simulink model "S_RS_B_Custom_Model"  (R2024b)
settings: Solver=ode23t  StartTime=0.0  StopTime=6*3600  MaxStep=0.03  RelTol=1e-6
model workspace (MAT data in the model file):
  C048A = [-4.646 -4.60016161616 -4.553 -4.506 -4.459 -4.41180808081 -4.36496969697 -4.31813131313 -4.27129292929 -4.22445454545 -4.17761616162 -4.13077777778 ... (100 elements, 100x1)]
  C25C = [-4.6365 -4.58998989899 -4.54347979798 -4.49604545455 -4.44945959596 -4.40294949495 -4.35593939394 -4.30893939394 -4.26241919192 -4.21540909091 -4.16848484848 -4.12155555556 ... (100 elements, 100x1)]
  C40C = [-4.693 -4.64635858586 -4.59905555556 -4.55133333333 -4.50411111111 -4.45679292929 -4.40916666667 -4.36194444444 -4.31472222222 -4.26727272727 -4.21977777778 -4.17244444444 ... (100 elements, 100x1)]
  C48A = [-4.565 -4.51971717172 -4.47343434343 -4.42715151515 -4.38086868687 -4.335 -4.289 -4.243 -4.19673737374 -4.15045454545 -4.10417171717 -4.058 ... (100 elements, 100x1)]
  C55C = [-4.736 -4.68873737374 -4.64097474747 -4.59321212121 -4.54544444444 -4.49718686869 -4.44942424242 -4.40166161616 -4.3538989899 -4.30613636364 -4.25837373737 -4.21061111111 ... (100 elements, 100x1)]
  C72A = [-4.552 -4.50695959596 -4.46091919192 -4.41487878788 -4.36983838384 -4.3237979798 -4.27775757576 -4.23171717172 -4.18567676768 -4.13963636364 -4.0935959596 -4.04755555556 ... (100 elements, 100x1)]
  C96A = [-4.554 -4.5084040404 -4.4625 -4.4165 -4.3705 -4.32467676768 -4.27863636364 -4.23257575758 -4.18651515152 -4.14045454545 -4.09439393939 -4.04838888889 ... (100 elements, 100x1)]
  I048A = [-0.48 -0.48 -0.48 -0.48 -0.48 -0.48 -0.48 -0.48 -0.48 -0.48 -0.48 -0.48 ... (100 elements, 100x1)]
  I48A = [-4.792 -4.792 -4.792 -4.792 -4.792 -4.792 -4.792 -4.792 -4.792 -4.792 -4.792 -4.792 ... (100 elements, 100x1)]
  I72A = [-7.19 -7.191 -7.191 -7.191 -7.191 -7.191 -7.191 -7.191 -7.191 -7.191 -7.191 -7.191 ... (100 elements, 100x1)]
  I96A = [-9.591 -9.591 -9.591 -9.591 -9.591 -9.591 -9.591 -9.591 -9.591 -9.591 -9.591 -9.591 ... (100 elements, 100x1)]
  Param : Simulink.Parameter (value not decoded)
  RT048 = [0 0 0 0 0 0 0 0 0 0 0 0 ... (100 elements, 100x1)]
  RT048A = [0 0 0 0 0 0 0 0 0 0 0 0 ... (100 elements, 100x1)]
  RT48A = [0 0.0119433061837 0.0174343602975 0.0201725097385 0.0218841166254 0.022368931384 0.0223984418475 0.0231362034367 0.0227462437396 0.0224237365306 0.0230708588388 0.0242533852717 ... (100 elements, 100x1)]
  RT72A = [0 0.0122979200993 0.0175935407475 0.020202020202 0.0216937838965 0.0225267555263 0.0230549129172 0.0237221330254 0.0239187873731 0.0241969128077 0.0252237294373 0.0266691388928 ... (100 elements, 100x1)]
  RT96A = [0 0.0106302309931 0.015521179894 0.0181246307302 0.0198249832282 0.0208391916243 0.0215479790081 0.0224110566619 0.0227069990911 0.0230234784504 0.0239687038248 0.0253072903996 ... (100 elements, 100x1)]
  SOC01C = [0 0.00986620401171 0.0200172191132 0.0301334481274 0.0402496771416 0.0504072146345 0.0604886575614 0.0705701004883 0.0806515434152 0.0907329863421 0.100814429269 0.110895872196 ... (100 elements, 100x1)]
  SOC15C = [0 0.00989464060642 0.0200089648684 0.0301232891303 0.0400179297367 0.0501322539987 0.0602465782606 0.0703609025226 0.0804752267845 0.0905895510465 0.100703875308 0.11081819957 ... (100 elements, 100x1)]
  SOC1C = [0 0.00991956807948 0.0200581942093 0.0301968203392 0.0403354464691 0.0503833515882 0.0604600219058 0.0705366922234 0.0806708929381 0.090809519068 0.100948145198 0.111062431544 ... (100 elements, 100x1)]
  SOC25C = [0 0.0100312953758 0.0200625907517 0.0302932266698 0.0403408614344 0.0503721568102 0.0605112921515 0.0706482489077 0.0806817228687 0.0908208582101 0.100941475578 0.111063182238 ... (100 elements, 100x1)]
  SOC2C = [0 0.0100122880097 0.020092226614 0.030193236715 0.040294246816 0.050356441002 0.0604663233122 0.0705806417269 0.0806949601416 0.0908092785563 0.100923596971 0.111025716098 ... (100 elements, 100x1)]
  SOC40C = [0 0.00993850716842 0.0200179937022 0.03018680304 0.04024907072 0.0503317857888 0.0604801477378 0.0705424154178 0.0806046830978 0.090715378804 0.100835760116 0.110921703719 ... (100 elements, 100x1)]
  SOC55C = [0 0.00997943966694 0.0200644536582 0.0301494676495 0.040235548048 0.0504250699563 0.0605100839476 0.0705950979388 0.0806801119301 0.0907651259214 0.100850139913 0.110935153904 ... (100 elements, 100x1)]
  T25C = [297.946805556 297.946193603 297.929952862 297.907583333 297.879161616 297.864882155 297.845863636 297.84875 297.844378788 297.852901515 297.87439899 297.893138889 ... (100 elements, 100x1)]
  T40C = [312.783611111 312.799016835 312.779327441 312.709037879 312.764760943 312.775969697 312.760472222 312.812088384 312.770179293 312.777401515 312.764757576 312.816768519 ... (100 elements, 100x1)]
  T55C = [327.602916667 327.628770202 327.629694444 327.60230303 327.617340909 327.627280303 327.630606061 327.639113636 327.603484848 327.641583333 327.626977273 327.647388889 ... (100 elements, 100x1)]
  V048A = [2.5 2.68851515152 2.80367676768 2.88551515152 2.951 3.00419191919 3.05003030303 3.09186868687 3.124 3.153 3.18438383838 3.21722222222 ... (100 elements, 100x1)]
  V25C = [2.4995 2.68887878788 2.80454040404 2.88553030303 2.95054040404 3.00379292929 3.04906060606 3.09057070707 3.13208080808 3.17309090909 3.21251515152 3.24794444444 ... (100 elements, 100x1)]
  V40C = [2.499 2.68894444444 2.80844444444 2.89090909091 2.95538888889 3.00911111111 3.05384848485 3.09348989899 3.13214646465 3.17127272727 3.21022222222 3.24738888889 ... (100 elements, 100x1)]
  V48A = [2.5 2.63128282828 2.72013131313 2.78884848485 2.84613131313 2.897 2.9426969697 2.981 3.015 3.04554545455 3.07382828283 3.101 ... (100 elements, 100x1)]
  V55C = [2.499 2.68891414141 2.80855050505 2.89028787879 2.95405050505 3.00636868687 3.05007575758 3.08772222222 3.12348989899 3.1595 3.19588888889 3.2315 ... (100 elements, 100x1)]
  V72A = [2.5 2.60008080808 2.67716161616 2.74024242424 2.795 2.8422020202 2.88424242424 2.92128282828 2.952 2.979 3.003 3.02544444444 ... (100 elements, 100x1)]
  V96A = [2.5 2.58656060606 2.65481313131 2.71168181818 2.76085858586 2.80432323232 2.84336363636 2.87692424242 2.90621717172 2.93218181818 2.9545 2.9745 ... (100 elements, 100x1)]
  t_CHG_25C = [18010 17847.8787879 17665.7575758 17483.6363636 17301.5151515 17119.3939394 16952.2727273 16770.1515152 16588.030303 16420.9090909 16238.7878788 16056.6666667 ... (100 elements, 100x1)]
  t_CHG_40C = [14605 14477.2727273 14329.5454545 14181.8181818 14049.0909091 13901.3636364 13768.6363636 13620.9090909 13473.1818182 13325.4545455 13177.7272727 13030 ... (100 elements, 100x1)]
  t_CHG_55C = [17190 17046.0606061 16872.1212121 16719.5454545 16554.2424242 16380.3030303 16206.3636364 16032.4242424 15858.4848485 15684.5454545 15510.6060606 15336.6666667 ... (100 elements, 100x1)]
libraries: BatteryEstimators x1
(part 2 of 2)

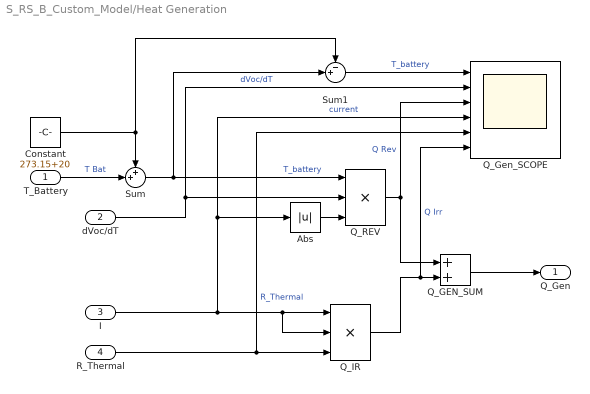
== system S_RS_B_Custom_Model/Heat Generation ==
  T_Battery : Inport
  dVoc/dT : Inport  Port=2
  I : Inport  Port=3
  R_Thermal : Inport  Port=4
  Abs : Abs  SaturateOnIntegerOverflow=off
  Constant : Constant  Value=273.15+20
  Q_GEN_SUM : Sum
  Q_Gen_SCOPE : Scope  NumInputPorts=6
  Q_IR : Product  Inputs=3
  Q_REV : Product  Inputs=3
  Sum : Sum  Inputs=++|
  Sum1 : Sum  Inputs=-+|
  Q_Gen : Outport
  wires:
  Q_REV/1 -> Q_GEN_SUM/1, Q_Gen_SCOPE/3  "Q Rev"
  I/1 -> Q_IR/2, Q_IR/1, Abs/1, Q_Gen_SCOPE/4  "current"
  R_Thermal/1 -> Q_IR/3, Q_Gen_SCOPE/5  "R_Thermal"
  Q_IR/1 -> Q_Gen_SCOPE/6, Q_GEN_SUM/2  "Q Irr"
  dVoc/dT/1 -> Q_REV/2, Q_Gen_SCOPE/2  "dVoc/dT"
  Q_GEN_SUM/1 -> Q_Gen/1
  Abs/1 -> Q_REV/3
  T_Battery/1 -> Sum/2  "T Bat"
  Constant/1 -> Sum1/1, Sum/1
  Sum/1 -> Sum1/2, Q_REV/1  "T_battery"
  Sum1/1 -> Q_Gen_SCOPE/1  "T_battery"

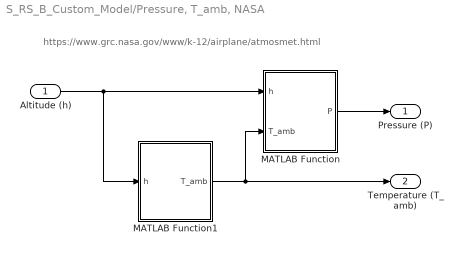
== system S_RS_B_Custom_Model/Pressure, T_amb, NASA ==
  note: https://www.grc.nasa.gov/www/k-12/airplane/atmosmet.html
  Altitude (h) : Inport
  MATLAB Function : MATLAB Function  TreatAsAtomicUnit=on
  MATLAB Function1 : MATLAB Function  TreatAsAtomicUnit=on
  Pressure (P) : Outport
  Temperature (T_amb) : Outport  Port=2
  wires:
  MATLAB Function1/1(T_amb) -> MATLAB Function/2(T_amb), Temperature (T_amb)/1
  MATLAB Function/1(P) -> Pressure (P)/1
  Altitude (h)/1 -> MATLAB Function/1(h), MATLAB Function1/1(h)

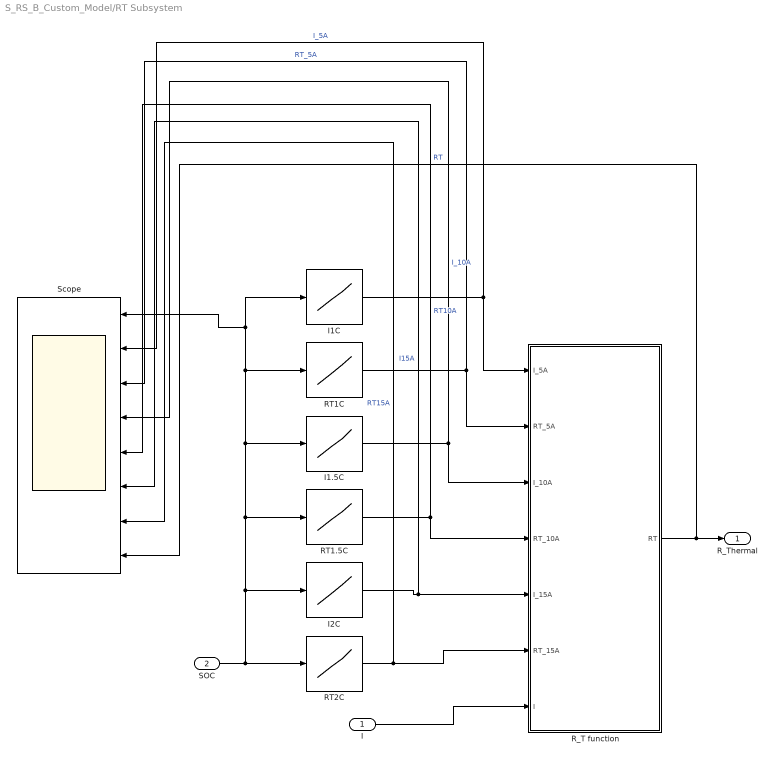
== system S_RS_B_Custom_Model/RT Subsystem ==
  I : Inport
  SOC : Inport  Port=2
  I1.5C : Lookup_n-D  NumberOfTableDimensions=1  BreakpointsForDimension1=SOC15C  Table=I72A  InternalRulePriority=Speed  RndMeth=Simplest
  I1C : Lookup_n-D  NumberOfTableDimensions=1  BreakpointsForDimension1=SOC1C  Table=I48A  InternalRulePriority=Speed  RndMeth=Simplest
  I2C : Lookup_n-D  NumberOfTableDimensions=1  BreakpointsForDimension1=SOC2C  Table=I96A  InternalRulePriority=Speed  RndMeth=Simplest
  RT1.5C : Lookup_n-D  NumberOfTableDimensions=1  BreakpointsForDimension1=SOC15C  Table=RT72A  InternalRulePriority=Speed  RndMeth=Simplest
  RT1C : Lookup_n-D  NumberOfTableDimensions=1  BreakpointsForDimension1=SOC1C  Table=RT48A  InternalRulePriority=Speed  RndMeth=Simplest
  RT2C : Lookup_n-D  NumberOfTableDimensions=1  BreakpointsForDimension1=SOC2C  Table=RT96A  InternalRulePriority=Speed  RndMeth=Simplest
  R_T function : MATLAB Function  TreatAsAtomicUnit=on
  Scope : Scope  NumInputPorts=8
  R_Thermal : Outport
  wires:
  R_T function/1(RT) -> Scope/8, R_Thermal/1  "RT"
  I/1 -> R_T function/7(I)
  SOC/1 -> RT1C/1, I1C/1, Scope/1, I1.5C/1, RT1.5C/1, I2C/1, RT2C/1
  I1C/1 -> R_T function/1(I_5A), Scope/2  "I_5A"
  RT1C/1 -> R_T function/2(RT_5A), Scope/3  "RT_5A"
  I1.5C/1 -> R_T function/3(I_10A), Scope/4  "I_10A"
  RT1.5C/1 -> R_T function/4(RT_10A), Scope/5  "RT10A"
  I2C/1 -> Scope/6, R_T function/5(I_15A)  "I15A"
  RT2C/1 -> Scope/7, R_T function/6(RT_15A)  "RT15A"

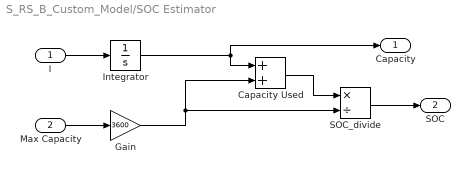
== system S_RS_B_Custom_Model/SOC Estimator ==
  I : Inport
  Max Capacity : Inport  Port=2
  Capacity Used : Sum
  Gain : Gain  Gain=3600
  Integrator : Integrator
  SOC_divide : Product  Inputs=*/
  Capacity : Outport
  SOC : Outport  Port=2
  wires:
  Capacity Used/1 -> SOC_divide/1
  SOC_divide/1 -> SOC/1
  I/1 -> Integrator/1
  Max Capacity/1 -> Gain/1
  Gain/1 -> SOC_divide/2, Capacity Used/2
  Integrator/1 -> Capacity Used/1, Capacity/1

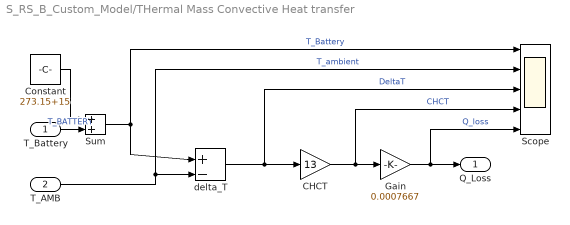
== system S_RS_B_Custom_Model/THermal Mass Convective Heat transfer ==
  T_Battery : Inport
  T_AMB : Inport  Port=2
  CHCT : Gain  Gain=13
  Constant : Constant  Value=273.15+15
  Gain : Gain  Gain=0.0007667
  Scope : Scope  NumInputPorts=5
  Sum : Sum  Inputs=+|+
  delta_T : Sum  Inputs=+|-
  Q_Loss : Outport
  wires:
  T_AMB/1 -> Scope/2, delta_T/2  "T_ambient"
  delta_T/1 -> Scope/3, CHCT/1  "DeltaT"
  CHCT/1 -> Scope/4, Gain/1  "CHCT"
  Gain/1 -> Scope/5, Q_Loss/1  "Q_loss"
  T_Battery/1 -> Sum/2  "T_BATTERY"
  Sum/1 -> delta_T/1, Scope/1  "T_Battery"
  Constant/1 -> Sum/1

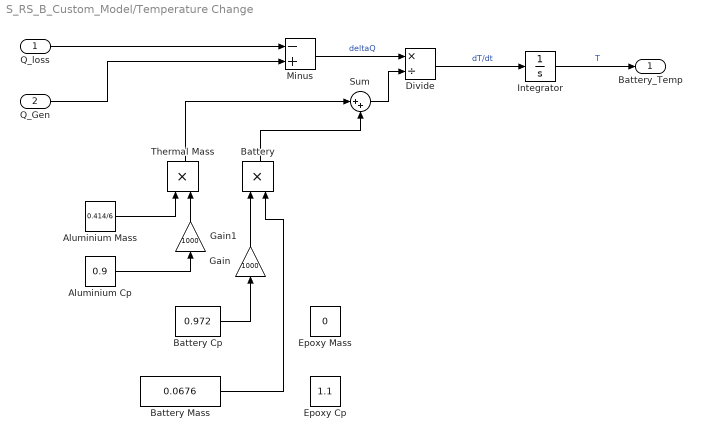
== system S_RS_B_Custom_Model/Temperature Change ==
  Q_loss : Inport
  Q_Gen : Inport  Port=2
  Aluminium Cp : Constant  Value=0.9  VectorParams1D=off
  Aluminium Mass : Constant  Value=0.414/6  VectorParams1D=off
  Battery : Product  OutDataTypeStr=double
  Battery Cp : Constant  Value=0.972  VectorParams1D=off
  Battery Mass : Constant  Value=0.0676  VectorParams1D=off
  Divide : Product  Inputs=*/
  Epoxy Cp : Constant  Value=1.1  VectorParams1D=off
  Epoxy Mass : Constant  Value=0  VectorParams1D=off
  Gain : Gain  Gain=1000
  Gain1 : Gain  Gain=1000
  Integrator : Integrator
  Minus : Sum  Inputs=-+
  Sum : Sum  Inputs=|++
  Thermal Mass : Product  OutDataTypeStr=double
  Battery_Temp : Outport
  wires:
  Integrator/1 -> Battery_Temp/1  "T"
  Battery/1 -> Sum/2
  Divide/1 -> Integrator/1  "dT/dt"
  Minus/1 -> Divide/1  "deltaQ"
  Sum/1 -> Divide/2
  Battery Cp/1 -> Gain/1
  Aluminium Cp/1 -> Gain1/1
  Aluminium Mass/1 -> Thermal Mass/1
  Q_loss/1 -> Minus/1
  Q_Gen/1 -> Minus/2
  Battery Mass/1 -> Battery/2
  Gain/1 -> Battery/1
  Thermal Mass/1 -> Sum/1
  Gain1/1 -> Thermal Mass/2

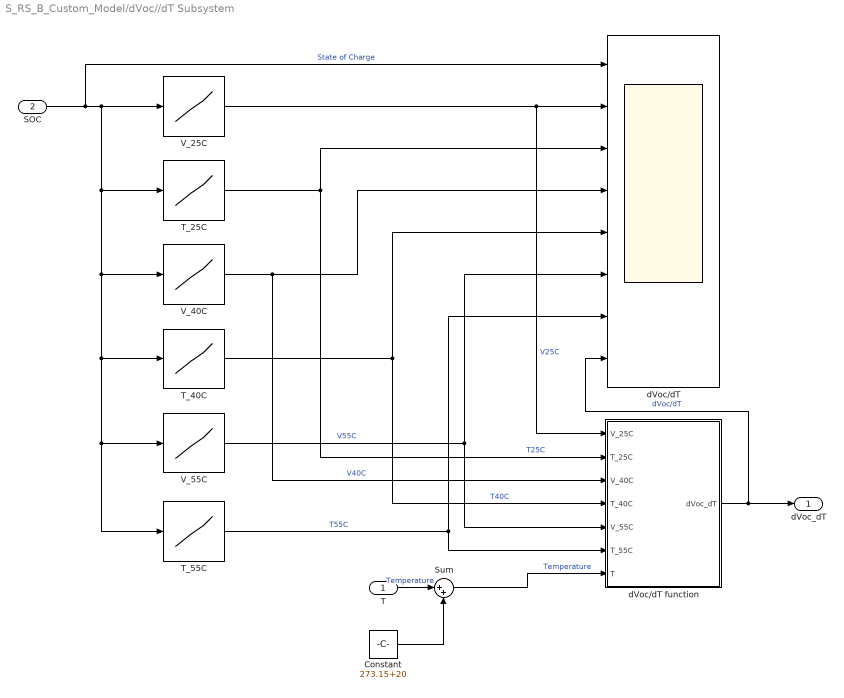
== system S_RS_B_Custom_Model/dVoc//dT Subsystem ==
  T : Inport
  SOC : Inport  Port=2
  Constant : Constant  Value=273.15+20
  Sum : Sum  Inputs=|++
  T_25C : Lookup_n-D  NumberOfTableDimensions=1  BreakpointsForDimension1=SOC25C  Table=T25C  InternalRulePriority=Speed  RndMeth=Simplest  SupportTunableSize=on
  T_40C : Lookup_n-D  NumberOfTableDimensions=1  BreakpointsForDimension1=SOC40C  Table=T40C  InternalRulePriority=Speed  RndMeth=Simplest  SupportTunableSize=on
  T_55C : Lookup_n-D  NumberOfTableDimensions=1  BreakpointsForDimension1=SOC55C  Table=T55C  InternalRulePriority=Speed  RndMeth=Simplest  SupportTunableSize=on
  V_25C : Lookup_n-D  NumberOfTableDimensions=1  BreakpointsForDimension1=SOC25C  Table=V25C  InternalRulePriority=Speed  RndMeth=Simplest  SupportTunableSize=on
  V_40C : Lookup_n-D  NumberOfTableDimensions=1  BreakpointsForDimension1=SOC40C  Table=V40C  InternalRulePriority=Speed  RndMeth=Simplest  SupportTunableSize=on
  V_55C : Lookup_n-D  NumberOfTableDimensions=1  BreakpointsForDimension1=SOC55C  Table=V55C  InternalRulePriority=Speed  RndMeth=Simplest  SupportTunableSize=on
  dVoc/dT : Scope  NumInputPorts=8
  dVoc/dT function : MATLAB Function  TreatAsAtomicUnit=on
  dVoc_dT : Outport
  wires:
  Sum/1 -> dVoc/dT function/7(T)  "Temperature"
  dVoc/dT function/1(dVoc_dT) -> dVoc/dT/8, dVoc_dT/1  "dVoc/dT"
  V_25C/1 -> dVoc/dT function/1(V_25C), dVoc/dT/2  "V25C"
  T_25C/1 -> dVoc/dT function/2(T_25C), dVoc/dT/3  "T25C"
  V_40C/1 -> dVoc/dT function/3(V_40C), dVoc/dT/4  "V40C"
  T_40C/1 -> dVoc/dT function/4(T_40C), dVoc/dT/5  "T40C"
  V_55C/1 -> dVoc/dT function/5(V_55C), dVoc/dT/6  "V55C"
  T_55C/1 -> dVoc/dT/7, dVoc/dT function/6(T_55C)  "T55C"
  SOC/1 -> dVoc/dT/1, T_55C/1, V_55C/1, T_40C/1, V_40C/1, T_25C/1, V_25C/1  "State of Charge"
  T/1 -> Sum/1  "Temperature"
  Constant/1 -> Sum/2

== matlab function S_RS_B_Custom_Model/RT Subsystem/R_T function ==
  data: I_5A input; RT_5A input; I_10A input; RT output; RT_10A input; I_15A input; RT_15A input; I input
function RT = fcn(I_5A,RT_5A, I_10A,RT_10A, I_15A,RT_15A, I)
    
    %Current Index
    a= I_5A;
    b= I_10A;
    c= I_15A;

    %Lagrange polynomial 
  
    Rt_1C = RT_5A .* (I-b) .* (I-c)  ./ ((a-b) .* (a-c) ); 
    Rt_2C = RT_10A .* (I-a) .* (I-c) ./ ((b-a) .* (b-c) );
    Rt_3C = RT_15A .* (I-a) .* (I-b) ./ ((c-a) .* (c-b) );

    RT = Rt_1C + Rt_2C + Rt_3C; 

end

== matlab function S_RS_B_Custom_Model/dVoc//dT Subsystem/dVoc//dT function ==
  data: V_25C input; T_25C input; V_40C input; T_40C input; V_55C input; T_55C input; T input; dVoc_dT output
function dVoc_dT = fcn(V_25C,T_25C, V_40C,T_40C, V_55C,T_55C,  T)

    dVoc_25C = V_25C .* (2*T - T_40C - T_55C) / ( (T_25C - T_40C ) * (T_25C - T_55C) ); 
    dVoc_40C = V_40C .* (2*T - T_25C - T_55C) / ( (T_40C - T_25C ) * (T_40C - T_55C ) ); 
    dVoc_55C = V_55C .* (2*T - T_25C - T_40C) / ( (T_55C - T_25C ) * (T_55C - T_40C ) );

    %Output
    dVoc_dT = double(dVoc_25C + dVoc_40C + dVoc_55C); 
    
end

== matlab function S_RS_B_Custom_Model/Cell Voltage/V function ==
  data: I_0_5A input; V_0_5A input; I_5A input; V_5A input; I_10A input; V output; V_10A input; I_15A input; V_15A input; I input
function V = fcn(I_0_5A,V_0_5A, I_5A,V_5A, I_10A,V_10A, I_15A,V_15A, I)
    

    a= I_0_5A;
    b= I_5A;
    c= I_10A;
    d= I_15A;

    %Lagrange polynomial 
    Rt_0_1C = V_0_5A .* (I-b) .*(I-c) .* (I-d) ./ ((a-b) .* (a-c) .* (a-d) );
    Rt_1C = V_5A .* (I-a) .* (I-c) .* (I-d) ./ ((b-a) .* (b-c) .* (b-d) ); 
    Rt_2C = V_10A .* (I-a) .* (I-b) .* (I-d) ./ ((c-a) .* (c-b) .* (c-d) );
    Rt_3C = V_15A .* (I-a) .* (I-b) .* (I-c) ./ ((d-a) .* (d-b) .* (d-c) );

    V = double( Rt_0_1C + Rt_1C + Rt_2C + Rt_3C ); 

end

== matlab function S_RS_B_Custom_Model/Pressure, T_amb, NASA/MATLAB Function ==
  data: h input; P output; T_amb input
function P = Pressure(h, T_amb)
    if h>=25000
        P = 2.488 * (T_amb/216.6).^(-11.388) *10^3 ;%Pressure, kPa
    elseif (h >= 11000) && (h<=25000)
        P = 22.65*exp(1.73-0.000157*h) ;%Pressure, kPa
    elseif h>= 11000 
        P=101.29*(T_amb/288.08).^(5.256) ;%Pressure, kPa 
    else 
        P=0; 
    end
end

== matlab function S_RS_B_Custom_Model/Pressure, T_amb, NASA/MATLAB Function1 ==
  data: h input; T_amb output
function T_amb = Temperature(h)
    if h>=25000
        T_amb =-131.21+0.00299*h + 273.15 ;%T_amb, kelvin
    elseif (h >= 11000) && (h<=25000)
        T_amb = -56.46 +273.15; %T_amb, kelvin
    elseif h>= 11000 
        T_amb = 15.04-0.00649*h + 273.15; %T_amb, kelvin 
    else 
        T_amb = 0;
    end
end
